simulink model "largeWaterPumpingNetwork"  (R2023b)
settings: Solver=VariableStepAuto  StartTime=0.0  StopTime=200  MaxStep=1  RelTol=1e-5  AbsTol=1e-5  EnableMultiTasking=on
InitFcn:
  | load("largescale_sample.mat")
undefined symbols (not defined in the file or in its folder): input_parameters
libraries: fl_lib x243, nesl_utility x162, SimscapeFluids_lib x129, sdl_lib x40
(part 2 of 12)

== system largeWaterPumpingNetwork/Subsystem 3 ==
  Bus Creator : BusCreator  Inputs=4
  Line 11 : Subsystem  mask{source_pressure=input_parameters.source_pressure_11, pump_speed=input_parameters.pump_speed_11, pipe1_length=input_parameters.pipe1_length_11, pipe2_length=input_parameters.pipe2_length_11, pipe2_ele=input_parameters.pipe2_ele_11}
      mask prompts: source_pressure "Source Pressure (atm)"; pump_speed "Pump Speed (rpm)"; pipe1_length "Pipe #1 Length (m)"; pipe2_length "Pipe #2 Length (m)"; pipe2_ele "PIpe #3 Elevation Gain (m)"
      settings: PortSchema="{\"entries\":[{\"content\":{\"sides\":[{\"content\":{},\"type\":\"ConnectorPlacement.EquallySpacedRectSide\",\"uuid\":\"b3564357-8f52-4949-91c1-42582344ea16\"},{\"content\":{\"connectorIds\":[\"RConn1\"],\"side\":\"RIGHT\"},\"type\":\"ConnectorPlacement.EquallySpacedRectSide\",\"uuid\":\"3df6ff4b-c089-47d9-9218-1d5835660c11\"},{\"content\":{\"connectorIds\":[\"Out1\"],\"side\":\"TOP\"},\"type\":\"ConnectorPlacement.EquallySpacedRectSide\",\"uuid\":\"76d061bd-6b93-4208-81e2-7b97871dfce4\"}]},\"type\":\"ConnectorPlacement.EquallySpacedConnector\",\"uuid\":\"90c8a33d-31fc-4de8-aabb-a154bae7a0ca\"}],\"packageUris\":[\"http://schema.mathworks.com/mf0/Connector/R2020b\"],\"version\":\"1.0\"}"
  Line 12 : Subsystem  mask{source_pressure=input_parameters.source_pressure_12, pump_speed=input_parameters.pump_speed_12, pipe1_length=input_parameters.pipe1_length_12, pipe2_length=input_parameters.pipe2_length_12, pipe2_ele=input_parameters.pipe2_ele_12}
      mask prompts: source_pressure "Source Pressure (atm)"; pump_speed "Pump Speed (rpm)"; pipe1_length "Pipe #1 Length (m)"; pipe2_length "Pipe #2 Length (m)"; pipe2_ele "PIpe #3 Elevation Gain (m)"
      settings: PortSchema="{\"entries\":[{\"content\":{\"sides\":[{\"content\":{},\"type\":\"ConnectorPlacement.EquallySpacedRectSide\",\"uuid\":\"b3564357-8f52-4949-91c1-42582344ea16\"},{\"content\":{\"connectorIds\":[\"RConn1\"],\"side\":\"RIGHT\"},\"type\":\"ConnectorPlacement.EquallySpacedRectSide\",\"uuid\":\"3df6ff4b-c089-47d9-9218-1d5835660c11\"},{\"content\":{\"connectorIds\":[\"Out1\"],\"side\":\"TOP\"},\"type\":\"ConnectorPlacement.EquallySpacedRectSide\",\"uuid\":\"76d061bd-6b93-4208-81e2-7b97871dfce4\"}]},\"type\":\"ConnectorPlacement.EquallySpacedConnector\",\"uuid\":\"90c8a33d-31fc-4de8-aabb-a154bae7a0ca\"}],\"packageUris\":[\"http://schema.mathworks.com/mf0/Connector/R2020b\"],\"version\":\"1.0\"}"
  Line 13 : Subsystem  mask{source_pressure=input_parameters.source_pressure_13, pump_speed=input_parameters.pump_speed_13, pipe1_length=input_parameters.pipe1_length_13, pipe2_length=input_parameters.pipe2_length_13, pipe2_ele=input_parameters.pipe2_ele_13}
      mask prompts: source_pressure "Source Pressure (atm)"; pump_speed "Pump Speed (rpm)"; pipe1_length "Pipe #1 Length (m)"; pipe2_length "Pipe #2 Length (m)"; pipe2_ele "PIpe #3 Elevation Gain (m)"
      settings: PortSchema="{\"entries\":[{\"content\":{\"sides\":[{\"content\":{},\"type\":\"ConnectorPlacement.EquallySpacedRectSide\",\"uuid\":\"b3564357-8f52-4949-91c1-42582344ea16\"},{\"content\":{\"connectorIds\":[\"RConn1\"],\"side\":\"RIGHT\"},\"type\":\"ConnectorPlacement.EquallySpacedRectSide\",\"uuid\":\"3df6ff4b-c089-47d9-9218-1d5835660c11\"},{\"content\":{\"connectorIds\":[\"Out1\"],\"side\":\"TOP\"},\"type\":\"ConnectorPlacement.EquallySpacedRectSide\",\"uuid\":\"76d061bd-6b93-4208-81e2-7b97871dfce4\"}]},\"type\":\"ConnectorPlacement.EquallySpacedConnector\",\"uuid\":\"90c8a33d-31fc-4de8-aabb-a154bae7a0ca\"}],\"packageUris\":[\"http://schema.mathworks.com/mf0/Connector/R2020b\"],\"version\":\"1.0\"}"
  Line 14 : Subsystem  mask{source_pressure=input_parameters.source_pressure_14, pump_speed=input_parameters.pump_speed_14, pipe1_length=input_parameters.pipe1_length_14, pipe2_length=input_parameters.pipe2_length_14, pipe2_ele=input_parameters.pipe2_ele_14}
      mask prompts: source_pressure "Source Pressure (atm)"; pump_speed "Pump Speed (rpm)"; pipe1_length "Pipe #1 Length (m)"; pipe2_length "Pipe #2 Length (m)"; pipe2_ele "PIpe #3 Elevation Gain (m)"
      settings: PortSchema="{\"entries\":[{\"content\":{\"sides\":[{\"content\":{},\"type\":\"ConnectorPlacement.EquallySpacedRectSide\",\"uuid\":\"b3564357-8f52-4949-91c1-42582344ea16\"},{\"content\":{\"connectorIds\":[\"RConn1\"],\"side\":\"RIGHT\"},\"type\":\"ConnectorPlacement.EquallySpacedRectSide\",\"uuid\":\"3df6ff4b-c089-47d9-9218-1d5835660c11\"},{\"content\":{\"connectorIds\":[\"Out1\"],\"side\":\"TOP\"},\"type\":\"ConnectorPlacement.EquallySpacedRectSide\",\"uuid\":\"76d061bd-6b93-4208-81e2-7b97871dfce4\"}]},\"type\":\"ConnectorPlacement.EquallySpacedConnector\",\"uuid\":\"90c8a33d-31fc-4de8-aabb-a154bae7a0ca\"}],\"packageUris\":[\"http://schema.mathworks.com/mf0/Connector/R2020b\"],\"version\":\"1.0\"}"
  Outflow : PMIOPort  Side=Left
  Inflow : PMIOPort  Port=2  Side=Right
  Sensor Signals : Outport
  wires:
  Bus Creator/1 -> Sensor Signals/1  "Sensor Signals"
  [Line11] -> Bus Creator/1  "Line11"
  Line 11/1(Sensor Signals) -> [Line11]
  Line 12/1(Sensor Signals) -> [Line12]
  Line 13/1(Sensor Signals) -> [Line13]
  Line 14/1(Sensor Signals) -> [Line14]
  [Line12] -> Bus Creator/2  "Line12"
  [Line13] -> Bus Creator/3  "Line13"
  [Line14] -> Bus Creator/4  "Line14"
  connections:
  Line 11/RConn1 -- Line 12/RConn1 -- Line 13/RConn1 -- Line 14/RConn1 -- Inflow/RConn1 -- Outflow/RConn1

== system largeWaterPumpingNetwork/Subsystem 4 ==
  Bus Creator : BusCreator  Inputs=5
  Line 15 : Subsystem  mask{source_pressure=input_parameters.source_pressure_15, pump_speed=input_parameters.pump_speed_15, pipe1_length=input_parameters.pipe1_length_15, pipe2_length=input_parameters.pipe2_length_15, pipe2_ele=input_parameters.pipe2_ele_15}
      mask prompts: source_pressure "Source Pressure (atm)"; pump_speed "Pump Speed (rpm)"; pipe1_length "Pipe #1 Length (m)"; pipe2_length "Pipe #2 Length (m)"; pipe2_ele "PIpe #3 Elevation Gain (m)"
      settings: PortSchema="{\"entries\":[{\"content\":{\"sides\":[{\"content\":{},\"type\":\"ConnectorPlacement.EquallySpacedRectSide\",\"uuid\":\"b3564357-8f52-4949-91c1-42582344ea16\"},{\"content\":{\"connectorIds\":[\"RConn1\"],\"side\":\"RIGHT\"},\"type\":\"ConnectorPlacement.EquallySpacedRectSide\",\"uuid\":\"3df6ff4b-c089-47d9-9218-1d5835660c11\"},{\"content\":{\"connectorIds\":[\"Out1\"],\"side\":\"TOP\"},\"type\":\"ConnectorPlacement.EquallySpacedRectSide\",\"uuid\":\"76d061bd-6b93-4208-81e2-7b97871dfce4\"}]},\"type\":\"ConnectorPlacement.EquallySpacedConnector\",\"uuid\":\"90c8a33d-31fc-4de8-aabb-a154bae7a0ca\"}],\"packageUris\":[\"http://schema.mathworks.com/mf0/Connector/R2020b\"],\"version\":\"1.0\"}"
  Line 16 : Subsystem  mask{source_pressure=input_parameters.source_pressure_16, pump_speed=input_parameters.pump_speed_16, pipe1_length=input_parameters.pipe1_length_16, pipe2_length=input_parameters.pipe2_length_16, pipe2_ele=input_parameters.pipe2_ele_16}
      mask prompts: source_pressure "Source Pressure (atm)"; pump_speed "Pump Speed (rpm)"; pipe1_length "Pipe #1 Length (m)"; pipe2_length "Pipe #2 Length (m)"; pipe2_ele "PIpe #3 Elevation Gain (m)"
      settings: PortSchema="{\"entries\":[{\"content\":{\"sides\":[{\"content\":{},\"type\":\"ConnectorPlacement.EquallySpacedRectSide\",\"uuid\":\"b3564357-8f52-4949-91c1-42582344ea16\"},{\"content\":{\"connectorIds\":[\"RConn1\"],\"side\":\"RIGHT\"},\"type\":\"ConnectorPlacement.EquallySpacedRectSide\",\"uuid\":\"3df6ff4b-c089-47d9-9218-1d5835660c11\"},{\"content\":{\"connectorIds\":[\"Out1\"],\"side\":\"TOP\"},\"type\":\"ConnectorPlacement.EquallySpacedRectSide\",\"uuid\":\"76d061bd-6b93-4208-81e2-7b97871dfce4\"}]},\"type\":\"ConnectorPlacement.EquallySpacedConnector\",\"uuid\":\"90c8a33d-31fc-4de8-aabb-a154bae7a0ca\"}],\"packageUris\":[\"http://schema.mathworks.com/mf0/Connector/R2020b\"],\"version\":\"1.0\"}"
  Line 17 : Subsystem  mask{source_pressure=input_parameters.source_pressure_17, pump_speed=input_parameters.pump_speed_17, pipe1_length=input_parameters.pipe1_length_17, pipe2_length=input_parameters.pipe2_length_17, pipe2_ele=input_parameters.pipe2_ele_17}
      mask prompts: source_pressure "Source Pressure (atm)"; pump_speed "Pump Speed (rpm)"; pipe1_length "Pipe #1 Length (m)"; pipe2_length "Pipe #2 Length (m)"; pipe2_ele "PIpe #3 Elevation Gain (m)"
      settings: PortSchema="{\"entries\":[{\"content\":{\"sides\":[{\"content\":{},\"type\":\"ConnectorPlacement.EquallySpacedRectSide\",\"uuid\":\"b3564357-8f52-4949-91c1-42582344ea16\"},{\"content\":{\"connectorIds\":[\"RConn1\"],\"side\":\"RIGHT\"},\"type\":\"ConnectorPlacement.EquallySpacedRectSide\",\"uuid\":\"3df6ff4b-c089-47d9-9218-1d5835660c11\"},{\"content\":{\"connectorIds\":[\"Out1\"],\"side\":\"TOP\"},\"type\":\"ConnectorPlacement.EquallySpacedRectSide\",\"uuid\":\"76d061bd-6b93-4208-81e2-7b97871dfce4\"}]},\"type\":\"ConnectorPlacement.EquallySpacedConnector\",\"uuid\":\"90c8a33d-31fc-4de8-aabb-a154bae7a0ca\"}],\"packageUris\":[\"http://schema.mathworks.com/mf0/Connector/R2020b\"],\"version\":\"1.0\"}"
  Line 18 : Subsystem  mask{source_pressure=input_parameters.source_pressure_18, pump_speed=input_parameters.pump_speed_18, pipe1_length=input_parameters.pipe1_length_18, pipe2_length=input_parameters.pipe2_length_18, pipe2_ele=input_parameters.pipe2_ele_18}
      mask prompts: source_pressure "Source Pressure (atm)"; pump_speed "Pump Speed (rpm)"; pipe1_length "Pipe #1 Length (m)"; pipe2_length "Pipe #2 Length (m)"; pipe2_ele "PIpe #3 Elevation Gain (m)"
      settings: PortSchema="{\"entries\":[{\"content\":{\"sides\":[{\"content\":{},\"type\":\"ConnectorPlacement.EquallySpacedRectSide\",\"uuid\":\"b3564357-8f52-4949-91c1-42582344ea16\"},{\"content\":{\"connectorIds\":[\"RConn1\"],\"side\":\"RIGHT\"},\"type\":\"ConnectorPlacement.EquallySpacedRectSide\",\"uuid\":\"3df6ff4b-c089-47d9-9218-1d5835660c11\"},{\"content\":{\"connectorIds\":[\"Out1\"],\"side\":\"TOP\"},\"type\":\"ConnectorPlacement.EquallySpacedRectSide\",\"uuid\":\"76d061bd-6b93-4208-81e2-7b97871dfce4\"}]},\"type\":\"ConnectorPlacement.EquallySpacedConnector\",\"uuid\":\"90c8a33d-31fc-4de8-aabb-a154bae7a0ca\"}],\"packageUris\":[\"http://schema.mathworks.com/mf0/Connector/R2020b\"],\"version\":\"1.0\"}"
  Line 19 : Subsystem  mask{source_pressure=input_parameters.source_pressure_19, pump_speed=input_parameters.pump_speed_19, pipe1_length=input_parameters.pipe1_length_19, pipe2_length=input_parameters.pipe2_length_19, pipe2_ele=input_parameters.pipe2_ele_19}
      mask prompts: source_pressure "Source Pressure (atm)"; pump_speed "Pump Speed (rpm)"; pipe1_length "Pipe #1 Length (m)"; pipe2_length "Pipe #2 Length (m)"; pipe2_ele "PIpe #3 Elevation Gain (m)"
      settings: PortSchema="{\"entries\":[{\"content\":{\"sides\":[{\"content\":{},\"type\":\"ConnectorPlacement.EquallySpacedRectSide\",\"uuid\":\"b3564357-8f52-4949-91c1-42582344ea16\"},{\"content\":{\"connectorIds\":[\"RConn1\"],\"side\":\"RIGHT\"},\"type\":\"ConnectorPlacement.EquallySpacedRectSide\",\"uuid\":\"3df6ff4b-c089-47d9-9218-1d5835660c11\"},{\"content\":{\"connectorIds\":[\"Out1\"],\"side\":\"TOP\"},\"type\":\"ConnectorPlacement.EquallySpacedRectSide\",\"uuid\":\"76d061bd-6b93-4208-81e2-7b97871dfce4\"}]},\"type\":\"ConnectorPlacement.EquallySpacedConnector\",\"uuid\":\"90c8a33d-31fc-4de8-aabb-a154bae7a0ca\"}],\"packageUris\":[\"http://schema.mathworks.com/mf0/Connector/R2020b\"],\"version\":\"1.0\"}"
  Outflow : PMIOPort  Side=Left
  Inflow : PMIOPort  Port=2  Side=Right
  Sensor Signals : Outport
  wires:
  Bus Creator/1 -> Sensor Signals/1  "Sensor Signals"
  [Line15] -> Bus Creator/1  "Line15"
  Line 15/1(Sensor Signals) -> [Line15]
  Line 16/1(Sensor Signals) -> [Line16]
  Line 17/1(Sensor Signals) -> [Line17]
  Line 18/1(Sensor Signals) -> [Line18]
  [Line16] -> Bus Creator/2  "Line16"
  [Line17] -> Bus Creator/3  "Line17"
  [Line18] -> Bus Creator/4  "Line18"
  Line 19/1(Sensor Signals) -> [Line19]
  [Line19] -> Bus Creator/5  "Line19"
  connections:
  Line 15/RConn1 -- Line 16/RConn1 -- Line 17/RConn1 -- Outflow/RConn1 -- Line 18/RConn1 -- Line 19/RConn1 -- Inflow/RConn1

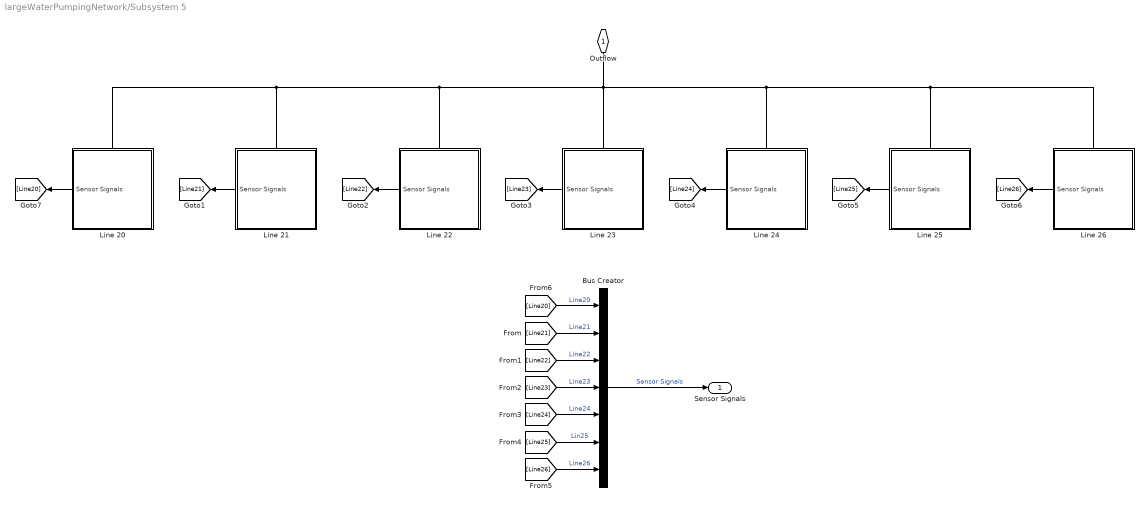
== system largeWaterPumpingNetwork/Subsystem 5 ==
  Bus Creator : BusCreator  Inputs=7
  Line 20 : Subsystem  mask{source_pressure=input_parameters.source_pressure_20, pump_speed=input_parameters.pump_speed_20, pipe1_length=input_parameters.pipe1_length_20, pipe2_length=input_parameters.pipe2_length_20, pipe2_ele=input_parameters.pipe2_ele_20}
      mask prompts: source_pressure "Source Pressure (atm)"; pump_speed "Pump Speed (rpm)"; pipe1_length "Pipe #1 Length (m)"; pipe2_length "Pipe #2 Length (m)"; pipe2_ele "PIpe #3 Elevation Gain (m)"
      settings: PortSchema="{\"entries\":[{\"content\":{\"sides\":[{\"content\":{},\"type\":\"ConnectorPlacement.EquallySpacedRectSide\",\"uuid\":\"b3564357-8f52-4949-91c1-42582344ea16\"},{\"content\":{\"connectorIds\":[\"RConn1\"],\"side\":\"RIGHT\"},\"type\":\"ConnectorPlacement.EquallySpacedRectSide\",\"uuid\":\"3df6ff4b-c089-47d9-9218-1d5835660c11\"},{\"content\":{\"connectorIds\":[\"Out1\"],\"side\":\"TOP\"},\"type\":\"ConnectorPlacement.EquallySpacedRectSide\",\"uuid\":\"76d061bd-6b93-4208-81e2-7b97871dfce4\"}]},\"type\":\"ConnectorPlacement.EquallySpacedConnector\",\"uuid\":\"90c8a33d-31fc-4de8-aabb-a154bae7a0ca\"}],\"packageUris\":[\"http://schema.mathworks.com/mf0/Connector/R2020b\"],\"version\":\"1.0\"}"
  Line 21 : Subsystem  mask{source_pressure=input_parameters.source_pressure_21, pump_speed=input_parameters.pump_speed_21, pipe1_length=input_parameters.pipe1_length_21, pipe2_length=input_parameters.pipe2_length_21, pipe2_ele=input_parameters.pipe2_ele_21}
      mask prompts: source_pressure "Source Pressure (atm)"; pump_speed "Pump Speed (rpm)"; pipe1_length "Pipe #1 Length (m)"; pipe2_length "Pipe #2 Length (m)"; pipe2_ele "PIpe #3 Elevation Gain (m)"
      settings: PortSchema="{\"entries\":[{\"content\":{\"sides\":[{\"content\":{},\"type\":\"ConnectorPlacement.EquallySpacedRectSide\",\"uuid\":\"b3564357-8f52-4949-91c1-42582344ea16\"},{\"content\":{\"connectorIds\":[\"RConn1\"],\"side\":\"RIGHT\"},\"type\":\"ConnectorPlacement.EquallySpacedRectSide\",\"uuid\":\"3df6ff4b-c089-47d9-9218-1d5835660c11\"},{\"content\":{\"connectorIds\":[\"Out1\"],\"side\":\"TOP\"},\"type\":\"ConnectorPlacement.EquallySpacedRectSide\",\"uuid\":\"76d061bd-6b93-4208-81e2-7b97871dfce4\"}]},\"type\":\"ConnectorPlacement.EquallySpacedConnector\",\"uuid\":\"90c8a33d-31fc-4de8-aabb-a154bae7a0ca\"}],\"packageUris\":[\"http://schema.mathworks.com/mf0/Connector/R2020b\"],\"version\":\"1.0\"}"
  Line 22 : Subsystem  mask{source_pressure=input_parameters.source_pressure_22, pump_speed=input_parameters.pump_speed_22, pipe1_length=input_parameters.pipe1_length_22, pipe2_length=input_parameters.pipe2_length_22, pipe2_ele=input_parameters.pipe2_ele_22}
      mask prompts: source_pressure "Source Pressure (atm)"; pump_speed "Pump Speed (rpm)"; pipe1_length "Pipe #1 Length (m)"; pipe2_length "Pipe #2 Length (m)"; pipe2_ele "PIpe #3 Elevation Gain (m)"
      settings: PortSchema="{\"entries\":[{\"content\":{\"sides\":[{\"content\":{},\"type\":\"ConnectorPlacement.EquallySpacedRectSide\",\"uuid\":\"b3564357-8f52-4949-91c1-42582344ea16\"},{\"content\":{\"connectorIds\":[\"RConn1\"],\"side\":\"RIGHT\"},\"type\":\"ConnectorPlacement.EquallySpacedRectSide\",\"uuid\":\"3df6ff4b-c089-47d9-9218-1d5835660c11\"},{\"content\":{\"connectorIds\":[\"Out1\"],\"side\":\"TOP\"},\"type\":\"ConnectorPlacement.EquallySpacedRectSide\",\"uuid\":\"76d061bd-6b93-4208-81e2-7b97871dfce4\"}]},\"type\":\"ConnectorPlacement.EquallySpacedConnector\",\"uuid\":\"90c8a33d-31fc-4de8-aabb-a154bae7a0ca\"}],\"packageUris\":[\"http://schema.mathworks.com/mf0/Connector/R2020b\"],\"version\":\"1.0\"}"
  Line 23 : Subsystem  mask{source_pressure=input_parameters.source_pressure_23, pump_speed=input_parameters.pump_speed_23, pipe1_length=input_parameters.pipe1_length_23, pipe2_length=input_parameters.pipe2_length_23, pipe2_ele=input_parameters.pipe2_ele_23}
      mask prompts: source_pressure "Source Pressure (atm)"; pump_speed "Pump Speed (rpm)"; pipe1_length "Pipe #1 Length (m)"; pipe2_length "Pipe #2 Length (m)"; pipe2_ele "PIpe #3 Elevation Gain (m)"
      settings: PortSchema="{\"entries\":[{\"content\":{\"sides\":[{\"content\":{},\"type\":\"ConnectorPlacement.EquallySpacedRectSide\",\"uuid\":\"b3564357-8f52-4949-91c1-42582344ea16\"},{\"content\":{\"connectorIds\":[\"RConn1\"],\"side\":\"RIGHT\"},\"type\":\"ConnectorPlacement.EquallySpacedRectSide\",\"uuid\":\"3df6ff4b-c089-47d9-9218-1d5835660c11\"},{\"content\":{\"connectorIds\":[\"Out1\"],\"side\":\"TOP\"},\"type\":\"ConnectorPlacement.EquallySpacedRectSide\",\"uuid\":\"76d061bd-6b93-4208-81e2-7b97871dfce4\"}]},\"type\":\"ConnectorPlacement.EquallySpacedConnector\",\"uuid\":\"90c8a33d-31fc-4de8-aabb-a154bae7a0ca\"}],\"packageUris\":[\"http://schema.mathworks.com/mf0/Connector/R2020b\"],\"version\":\"1.0\"}"
  Line 24 : Subsystem  mask{source_pressure=input_parameters.source_pressure_24, pump_speed=input_parameters.pump_speed_24, pipe1_length=input_parameters.pipe1_length_24, pipe2_length=input_parameters.pipe2_length_24, pipe2_ele=input_parameters.pipe2_ele_24}
      mask prompts: source_pressure "Source Pressure (atm)"; pump_speed "Pump Speed (rpm)"; pipe1_length "Pipe #1 Length (m)"; pipe2_length "Pipe #2 Length (m)"; pipe2_ele "PIpe #3 Elevation Gain (m)"
      settings: PortSchema="{\"entries\":[{\"content\":{\"sides\":[{\"content\":{},\"type\":\"ConnectorPlacement.EquallySpacedRectSide\",\"uuid\":\"b3564357-8f52-4949-91c1-42582344ea16\"},{\"content\":{\"connectorIds\":[\"RConn1\"],\"side\":\"RIGHT\"},\"type\":\"ConnectorPlacement.EquallySpacedRectSide\",\"uuid\":\"3df6ff4b-c089-47d9-9218-1d5835660c11\"},{\"content\":{\"connectorIds\":[\"Out1\"],\"side\":\"TOP\"},\"type\":\"ConnectorPlacement.EquallySpacedRectSide\",\"uuid\":\"76d061bd-6b93-4208-81e2-7b97871dfce4\"}]},\"type\":\"ConnectorPlacement.EquallySpacedConnector\",\"uuid\":\"90c8a33d-31fc-4de8-aabb-a154bae7a0ca\"}],\"packageUris\":[\"http://schema.mathworks.com/mf0/Connector/R2020b\"],\"version\":\"1.0\"}"
  Line 25 : Subsystem  mask{source_pressure=input_parameters.source_pressure_25, pump_speed=input_parameters.pump_speed_25, pipe1_length=input_parameters.pipe1_length_25, pipe2_length=input_parameters.pipe2_length_25, pipe2_ele=input_parameters.pipe2_ele_25}
      mask prompts: source_pressure "Source Pressure (atm)"; pump_speed "Pump Speed (rpm)"; pipe1_length "Pipe #1 Length (m)"; pipe2_length "Pipe #2 Length (m)"; pipe2_ele "PIpe #3 Elevation Gain (m)"
      settings: PortSchema="{\"entries\":[{\"content\":{\"sides\":[{\"content\":{},\"type\":\"ConnectorPlacement.EquallySpacedRectSide\",\"uuid\":\"b3564357-8f52-4949-91c1-42582344ea16\"},{\"content\":{\"connectorIds\":[\"RConn1\"],\"side\":\"RIGHT\"},\"type\":\"ConnectorPlacement.EquallySpacedRectSide\",\"uuid\":\"3df6ff4b-c089-47d9-9218-1d5835660c11\"},{\"content\":{\"connectorIds\":[\"Out1\"],\"side\":\"TOP\"},\"type\":\"ConnectorPlacement.EquallySpacedRectSide\",\"uuid\":\"76d061bd-6b93-4208-81e2-7b97871dfce4\"}]},\"type\":\"ConnectorPlacement.EquallySpacedConnector\",\"uuid\":\"90c8a33d-31fc-4de8-aabb-a154bae7a0ca\"}],\"packageUris\":[\"http://schema.mathworks.com/mf0/Connector/R2020b\"],\"version\":\"1.0\"}"
  Line 26 : Subsystem  mask{source_pressure=input_parameters.source_pressure_26, pump_speed=input_parameters.pump_speed_26, pipe1_length=input_parameters.pipe1_length_26, pipe2_length=input_parameters.pipe2_length_26, pipe2_ele=input_parameters.pipe2_ele_26}
      mask prompts: source_pressure "Source Pressure (atm)"; pump_speed "Pump Speed (rpm)"; pipe1_length "Pipe #1 Length (m)"; pipe2_length "Pipe #2 Length (m)"; pipe2_ele "PIpe #3 Elevation Gain (m)"
      settings: PortSchema="{\"entries\":[{\"content\":{\"sides\":[{\"content\":{},\"type\":\"ConnectorPlacement.EquallySpacedRectSide\",\"uuid\":\"b3564357-8f52-4949-91c1-42582344ea16\"},{\"content\":{\"connectorIds\":[\"RConn1\"],\"side\":\"RIGHT\"},\"type\":\"ConnectorPlacement.EquallySpacedRectSide\",\"uuid\":\"3df6ff4b-c089-47d9-9218-1d5835660c11\"},{\"content\":{\"connectorIds\":[\"Out1\"],\"side\":\"TOP\"},\"type\":\"ConnectorPlacement.EquallySpacedRectSide\",\"uuid\":\"76d061bd-6b93-4208-81e2-7b97871dfce4\"}]},\"type\":\"ConnectorPlacement.EquallySpacedConnector\",\"uuid\":\"90c8a33d-31fc-4de8-aabb-a154bae7a0ca\"}],\"packageUris\":[\"http://schema.mathworks.com/mf0/Connector/R2020b\"],\"version\":\"1.0\"}"
  Outflow : PMIOPort  Side=Left
  Sensor Signals : Outport
  wires:
  Bus Creator/1 -> Sensor Signals/1  "Sensor Signals"
  [Line21] -> Bus Creator/2  "Line21"
  Line 21/1(Sensor Signals) -> [Line21]
  Line 22/1(Sensor Signals) -> [Line22]
  Line 23/1(Sensor Signals) -> [Line23]
  Line 24/1(Sensor Signals) -> [Line24]
  [Line22] -> Bus Creator/3  "Line22"
  [Line23] -> Bus Creator/4  "Line23"
  [Line24] -> Bus Creator/5  "Line24"
  Line 25/1(Sensor Signals) -> [Line25]
  Line 26/1(Sensor Signals) -> [Line26]
  [Line25] -> Bus Creator/6  "Lin25"
  [Line26] -> Bus Creator/7  "Line26"
  Line 20/1(Sensor Signals) -> [Line20]
  [Line20] -> Bus Creator/1  "Line20"
  connections:
  Line 20/RConn1 -- Line 21/RConn1 -- Line 22/RConn1 -- Line 23/RConn1 -- Line 24/RConn1 -- Line 25/RConn1 -- Line 26/RConn1 -- Outflow/RConn1

== system largeWaterPumpingNetwork/Subsystem 6 ==
  Bus Creator : BusCreator  Inputs=4
  Line 27 : Subsystem  mask{source_pressure=input_parameters.source_pressure_27, pump_speed=input_parameters.pump_speed_27, pipe1_length=input_parameters.pipe1_length_27, pipe2_length=input_parameters.pipe2_length_27, pipe2_ele=input_parameters.pipe2_ele_27}
      mask prompts: source_pressure "Source Pressure (atm)"; pump_speed "Pump Speed (rpm)"; pipe1_length "Pipe #1 Length (m)"; pipe2_length "Pipe #2 Length (m)"; pipe2_ele "PIpe #3 Elevation Gain (m)"
      settings: PortSchema="{\"entries\":[{\"content\":{\"sides\":[{\"content\":{},\"type\":\"ConnectorPlacement.EquallySpacedRectSide\",\"uuid\":\"b3564357-8f52-4949-91c1-42582344ea16\"},{\"content\":{\"connectorIds\":[\"RConn1\"],\"side\":\"RIGHT\"},\"type\":\"ConnectorPlacement.EquallySpacedRectSide\",\"uuid\":\"3df6ff4b-c089-47d9-9218-1d5835660c11\"},{\"content\":{\"connectorIds\":[\"Out1\"],\"side\":\"TOP\"},\"type\":\"ConnectorPlacement.EquallySpacedRectSide\",\"uuid\":\"76d061bd-6b93-4208-81e2-7b97871dfce4\"}]},\"type\":\"ConnectorPlacement.EquallySpacedConnector\",\"uuid\":\"90c8a33d-31fc-4de8-aabb-a154bae7a0ca\"}],\"packageUris\":[\"http://schema.mathworks.com/mf0/Connector/R2020b\"],\"version\":\"1.0\"}"
  Line 28 : Subsystem  mask{source_pressure=input_parameters.source_pressure_28, pump_speed=input_parameters.pump_speed_28, pipe1_length=input_parameters.pipe1_length_28, pipe2_length=input_parameters.pipe2_length_28, pipe2_ele=input_parameters.pipe2_ele_28}
      mask prompts: source_pressure "Source Pressure (atm)"; pump_speed "Pump Speed (rpm)"; pipe1_length "Pipe #1 Length (m)"; pipe2_length "Pipe #2 Length (m)"; pipe2_ele "PIpe #3 Elevation Gain (m)"
      settings: PortSchema="{\"entries\":[{\"content\":{\"sides\":[{\"content\":{},\"type\":\"ConnectorPlacement.EquallySpacedRectSide\",\"uuid\":\"b3564357-8f52-4949-91c1-42582344ea16\"},{\"content\":{\"connectorIds\":[\"RConn1\"],\"side\":\"RIGHT\"},\"type\":\"ConnectorPlacement.EquallySpacedRectSide\",\"uuid\":\"3df6ff4b-c089-47d9-9218-1d5835660c11\"},{\"content\":{\"connectorIds\":[\"Out1\"],\"side\":\"TOP\"},\"type\":\"ConnectorPlacement.EquallySpacedRectSide\",\"uuid\":\"76d061bd-6b93-4208-81e2-7b97871dfce4\"}]},\"type\":\"ConnectorPlacement.EquallySpacedConnector\",\"uuid\":\"90c8a33d-31fc-4de8-aabb-a154bae7a0ca\"}],\"packageUris\":[\"http://schema.mathworks.com/mf0/Connector/R2020b\"],\"version\":\"1.0\"}"
  Line 29 : Subsystem  mask{source_pressure=input_parameters.source_pressure_29, pump_speed=input_parameters.pump_speed_29, pipe1_length=input_parameters.pipe1_length_29, pipe2_length=input_parameters.pipe2_length_29, pipe2_ele=input_parameters.pipe2_ele_29}
      mask prompts: source_pressure "Source Pressure (atm)"; pump_speed "Pump Speed (rpm)"; pipe1_length "Pipe #1 Length (m)"; pipe2_length "Pipe #2 Length (m)"; pipe2_ele "PIpe #3 Elevation Gain (m)"
      settings: PortSchema="{\"entries\":[{\"content\":{\"sides\":[{\"content\":{},\"type\":\"ConnectorPlacement.EquallySpacedRectSide\",\"uuid\":\"b3564357-8f52-4949-91c1-42582344ea16\"},{\"content\":{\"connectorIds\":[\"RConn1\"],\"side\":\"RIGHT\"},\"type\":\"ConnectorPlacement.EquallySpacedRectSide\",\"uuid\":\"3df6ff4b-c089-47d9-9218-1d5835660c11\"},{\"content\":{\"connectorIds\":[\"Out1\"],\"side\":\"TOP\"},\"type\":\"ConnectorPlacement.EquallySpacedRectSide\",\"uuid\":\"76d061bd-6b93-4208-81e2-7b97871dfce4\"}]},\"type\":\"ConnectorPlacement.EquallySpacedConnector\",\"uuid\":\"90c8a33d-31fc-4de8-aabb-a154bae7a0ca\"}],\"packageUris\":[\"http://schema.mathworks.com/mf0/Connector/R2020b\"],\"version\":\"1.0\"}"
  Line 30 : Subsystem  mask{source_pressure=input_parameters.source_pressure_30, pump_speed=input_parameters.pump_speed_30, pipe1_length=input_parameters.pipe1_length_30, pipe2_length=input_parameters.pipe2_length_30, pipe2_ele=input_parameters.pipe2_ele_30}
      mask prompts: source_pressure "Source Pressure (atm)"; pump_speed "Pump Speed (rpm)"; pipe1_length "Pipe #1 Length (m)"; pipe2_length "Pipe #2 Length (m)"; pipe2_ele "PIpe #3 Elevation Gain (m)"
      settings: PortSchema="{\"entries\":[{\"content\":{\"sides\":[{\"content\":{},\"type\":\"ConnectorPlacement.EquallySpacedRectSide\",\"uuid\":\"b3564357-8f52-4949-91c1-42582344ea16\"},{\"content\":{\"connectorIds\":[\"RConn1\"],\"side\":\"RIGHT\"},\"type\":\"ConnectorPlacement.EquallySpacedRectSide\",\"uuid\":\"3df6ff4b-c089-47d9-9218-1d5835660c11\"},{\"content\":{\"connectorIds\":[\"Out1\"],\"side\":\"TOP\"},\"type\":\"ConnectorPlacement.EquallySpacedRectSide\",\"uuid\":\"76d061bd-6b93-4208-81e2-7b97871dfce4\"}]},\"type\":\"ConnectorPlacement.EquallySpacedConnector\",\"uuid\":\"90c8a33d-31fc-4de8-aabb-a154bae7a0ca\"}],\"packageUris\":[\"http://schema.mathworks.com/mf0/Connector/R2020b\"],\"version\":\"1.0\"}"
  Outflow : PMIOPort  Side=Left
  Sensor Signals : Outport
  wires:
  Bus Creator/1 -> Sensor Signals/1  "Sensor Signals"
  [Line27] -> Bus Creator/1  "Line27"
  Line 27/1(Sensor Signals) -> [Line27]
  Line 28/1(Sensor Signals) -> [Line28]
  Line 29/1(Sensor Signals) -> [Line29]
  Line 30/1(Sensor Signals) -> [Line30]
  [Line28] -> Bus Creator/2  "Line28"
  [Line29] -> Bus Creator/3  "Line29"
  [Line30] -> Bus Creator/4  "Line30"
  connections:
  Line 27/RConn1 -- Line 28/RConn1 -- Line 29/RConn1 -- Line 30/RConn1 -- Outflow/RConn1

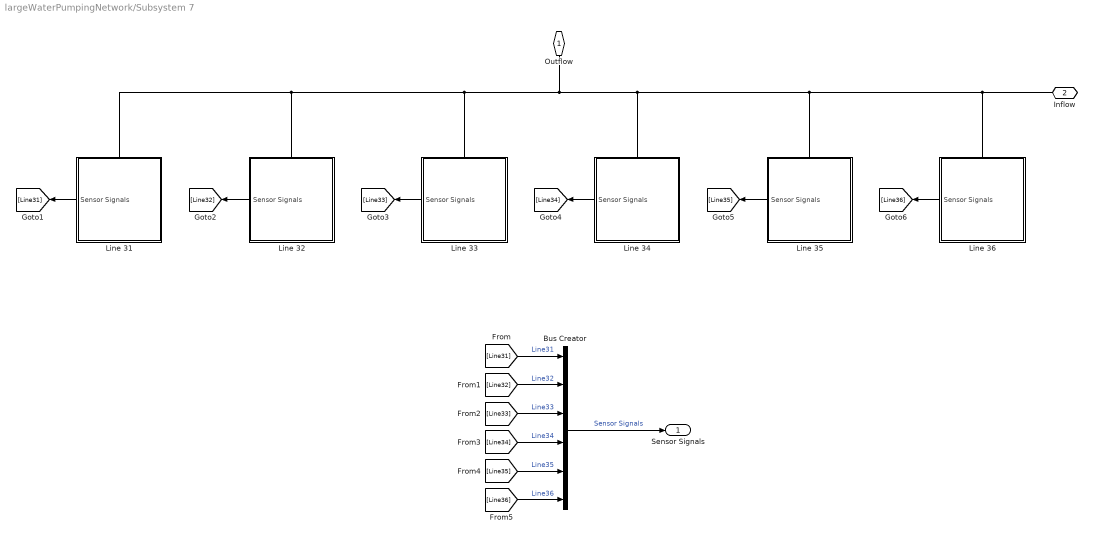
== system largeWaterPumpingNetwork/Subsystem 7 ==
  Bus Creator : BusCreator  Inputs=6
  Line 31 : Subsystem  mask{source_pressure=input_parameters.source_pressure_31, pump_speed=input_parameters.pump_speed_31, pipe1_length=input_parameters.pipe1_length_31, pipe2_length=input_parameters.pipe2_length_31, pipe2_ele=input_parameters.pipe2_ele_31}
      mask prompts: source_pressure "Source Pressure (atm)"; pump_speed "Pump Speed (rpm)"; pipe1_length "Pipe #1 Length (m)"; pipe2_length "Pipe #2 Length (m)"; pipe2_ele "PIpe #3 Elevation Gain (m)"
      settings: PortSchema="{\"entries\":[{\"content\":{\"sides\":[{\"content\":{},\"type\":\"ConnectorPlacement.EquallySpacedRectSide\",\"uuid\":\"b3564357-8f52-4949-91c1-42582344ea16\"},{\"content\":{\"connectorIds\":[\"RConn1\"],\"side\":\"RIGHT\"},\"type\":\"ConnectorPlacement.EquallySpacedRectSide\",\"uuid\":\"3df6ff4b-c089-47d9-9218-1d5835660c11\"},{\"content\":{\"connectorIds\":[\"Out1\"],\"side\":\"TOP\"},\"type\":\"ConnectorPlacement.EquallySpacedRectSide\",\"uuid\":\"76d061bd-6b93-4208-81e2-7b97871dfce4\"}]},\"type\":\"ConnectorPlacement.EquallySpacedConnector\",\"uuid\":\"90c8a33d-31fc-4de8-aabb-a154bae7a0ca\"}],\"packageUris\":[\"http://schema.mathworks.com/mf0/Connector/R2020b\"],\"version\":\"1.0\"}"
  Line 32 : Subsystem  mask{source_pressure=input_parameters.source_pressure_32, pump_speed=input_parameters.pump_speed_32, pipe1_length=input_parameters.pipe1_length_32, pipe2_length=input_parameters.pipe2_length_32, pipe2_ele=input_parameters.pipe2_ele_32}
      mask prompts: source_pressure "Source Pressure (atm)"; pump_speed "Pump Speed (rpm)"; pipe1_length "Pipe #1 Length (m)"; pipe2_length "Pipe #2 Length (m)"; pipe2_ele "PIpe #3 Elevation Gain (m)"
      settings: PortSchema="{\"entries\":[{\"content\":{\"sides\":[{\"content\":{},\"type\":\"ConnectorPlacement.EquallySpacedRectSide\",\"uuid\":\"b3564357-8f52-4949-91c1-42582344ea16\"},{\"content\":{\"connectorIds\":[\"RConn1\"],\"side\":\"RIGHT\"},\"type\":\"ConnectorPlacement.EquallySpacedRectSide\",\"uuid\":\"3df6ff4b-c089-47d9-9218-1d5835660c11\"},{\"content\":{\"connectorIds\":[\"Out1\"],\"side\":\"TOP\"},\"type\":\"ConnectorPlacement.EquallySpacedRectSide\",\"uuid\":\"76d061bd-6b93-4208-81e2-7b97871dfce4\"}]},\"type\":\"ConnectorPlacement.EquallySpacedConnector\",\"uuid\":\"90c8a33d-31fc-4de8-aabb-a154bae7a0ca\"}],\"packageUris\":[\"http://schema.mathworks.com/mf0/Connector/R2020b\"],\"version\":\"1.0\"}"
  Line 33 : Subsystem  mask{source_pressure=input_parameters.source_pressure_33, pump_speed=input_parameters.pump_speed_33, pipe1_length=input_parameters.pipe1_length_33, pipe2_length=input_parameters.pipe2_length_33, pipe2_ele=input_parameters.pipe2_ele_33}
      mask prompts: source_pressure "Source Pressure (atm)"; pump_speed "Pump Speed (rpm)"; pipe1_length "Pipe #1 Length (m)"; pipe2_length "Pipe #2 Length (m)"; pipe2_ele "PIpe #3 Elevation Gain (m)"
      settings: PortSchema="{\"entries\":[{\"content\":{\"sides\":[{\"content\":{},\"type\":\"ConnectorPlacement.EquallySpacedRectSide\",\"uuid\":\"b3564357-8f52-4949-91c1-42582344ea16\"},{\"content\":{\"connectorIds\":[\"RConn1\"],\"side\":\"RIGHT\"},\"type\":\"ConnectorPlacement.EquallySpacedRectSide\",\"uuid\":\"3df6ff4b-c089-47d9-9218-1d5835660c11\"},{\"content\":{\"connectorIds\":[\"Out1\"],\"side\":\"TOP\"},\"type\":\"ConnectorPlacement.EquallySpacedRectSide\",\"uuid\":\"76d061bd-6b93-4208-81e2-7b97871dfce4\"}]},\"type\":\"ConnectorPlacement.EquallySpacedConnector\",\"uuid\":\"90c8a33d-31fc-4de8-aabb-a154bae7a0ca\"}],\"packageUris\":[\"http://schema.mathworks.com/mf0/Connector/R2020b\"],\"version\":\"1.0\"}"
  Line 34 : Subsystem  mask{source_pressure=input_parameters.source_pressure_34, pump_speed=input_parameters.pump_speed_34, pipe1_length=input_parameters.pipe1_length_34, pipe2_length=input_parameters.pipe2_length_34, pipe2_ele=input_parameters.pipe2_ele_34}
      mask prompts: source_pressure "Source Pressure (atm)"; pump_speed "Pump Speed (rpm)"; pipe1_length "Pipe #1 Length (m)"; pipe2_length "Pipe #2 Length (m)"; pipe2_ele "PIpe #3 Elevation Gain (m)"
      settings: PortSchema="{\"entries\":[{\"content\":{\"sides\":[{\"content\":{},\"type\":\"ConnectorPlacement.EquallySpacedRectSide\",\"uuid\":\"b3564357-8f52-4949-91c1-42582344ea16\"},{\"content\":{\"connectorIds\":[\"RConn1\"],\"side\":\"RIGHT\"},\"type\":\"ConnectorPlacement.EquallySpacedRectSide\",\"uuid\":\"3df6ff4b-c089-47d9-9218-1d5835660c11\"},{\"content\":{\"connectorIds\":[\"Out1\"],\"side\":\"TOP\"},\"type\":\"ConnectorPlacement.EquallySpacedRectSide\",\"uuid\":\"76d061bd-6b93-4208-81e2-7b97871dfce4\"}]},\"type\":\"ConnectorPlacement.EquallySpacedConnector\",\"uuid\":\"90c8a33d-31fc-4de8-aabb-a154bae7a0ca\"}],\"packageUris\":[\"http://schema.mathworks.com/mf0/Connector/R2020b\"],\"version\":\"1.0\"}"
  Line 35 : Subsystem  mask{source_pressure=input_parameters.source_pressure_35, pump_speed=input_parameters.pump_speed_35, pipe1_length=input_parameters.pipe1_length_35, pipe2_length=input_parameters.pipe2_length_35, pipe2_ele=input_parameters.pipe2_ele_35}
      mask prompts: source_pressure "Source Pressure (atm)"; pump_speed "Pump Speed (rpm)"; pipe1_length "Pipe #1 Length (m)"; pipe2_length "Pipe #2 Length (m)"; pipe2_ele "PIpe #3 Elevation Gain (m)"
      settings: PortSchema="{\"entries\":[{\"content\":{\"sides\":[{\"content\":{},\"type\":\"ConnectorPlacement.EquallySpacedRectSide\",\"uuid\":\"b3564357-8f52-4949-91c1-42582344ea16\"},{\"content\":{\"connectorIds\":[\"RConn1\"],\"side\":\"RIGHT\"},\"type\":\"ConnectorPlacement.EquallySpacedRectSide\",\"uuid\":\"3df6ff4b-c089-47d9-9218-1d5835660c11\"},{\"content\":{\"connectorIds\":[\"Out1\"],\"side\":\"TOP\"},\"type\":\"ConnectorPlacement.EquallySpacedRectSide\",\"uuid\":\"76d061bd-6b93-4208-81e2-7b97871dfce4\"}]},\"type\":\"ConnectorPlacement.EquallySpacedConnector\",\"uuid\":\"90c8a33d-31fc-4de8-aabb-a154bae7a0ca\"}],\"packageUris\":[\"http://schema.mathworks.com/mf0/Connector/R2020b\"],\"version\":\"1.0\"}"
  Line 36 : Subsystem  mask{source_pressure=input_parameters.source_pressure_36, pump_speed=input_parameters.pump_speed_36, pipe1_length=input_parameters.pipe1_length_36, pipe2_length=input_parameters.pipe2_length_36, pipe2_ele=input_parameters.pipe2_ele_36}
      mask prompts: source_pressure "Source Pressure (atm)"; pump_speed "Pump Speed (rpm)"; pipe1_length "Pipe #1 Length (m)"; pipe2_length "Pipe #2 Length (m)"; pipe2_ele "PIpe #3 Elevation Gain (m)"
      settings: PortSchema="{\"entries\":[{\"content\":{\"sides\":[{\"content\":{},\"type\":\"ConnectorPlacement.EquallySpacedRectSide\",\"uuid\":\"b3564357-8f52-4949-91c1-42582344ea16\"},{\"content\":{\"connectorIds\":[\"RConn1\"],\"side\":\"RIGHT\"},\"type\":\"ConnectorPlacement.EquallySpacedRectSide\",\"uuid\":\"3df6ff4b-c089-47d9-9218-1d5835660c11\"},{\"content\":{\"connectorIds\":[\"Out1\"],\"side\":\"TOP\"},\"type\":\"ConnectorPlacement.EquallySpacedRectSide\",\"uuid\":\"76d061bd-6b93-4208-81e2-7b97871dfce4\"}]},\"type\":\"ConnectorPlacement.EquallySpacedConnector\",\"uuid\":\"90c8a33d-31fc-4de8-aabb-a154bae7a0ca\"}],\"packageUris\":[\"http://schema.mathworks.com/mf0/Connector/R2020b\"],\"version\":\"1.0\"}"
  Outflow : PMIOPort  Side=Left
  Inflow : PMIOPort  Port=2  Side=Right
  Sensor Signals : Outport
  wires:
  Bus Creator/1 -> Sensor Signals/1  "Sensor Signals"
  [Line31] -> Bus Creator/1  "Line31"
  Line 31/1(Sensor Signals) -> [Line31]
  Line 32/1(Sensor Signals) -> [Line32]
  Line 33/1(Sensor Signals) -> [Line33]
  Line 34/1(Sensor Signals) -> [Line34]
  [Line32] -> Bus Creator/2  "Line32"
  [Line33] -> Bus Creator/3  "Line33"
  [Line34] -> Bus Creator/4  "Line34"
  Line 35/1(Sensor Signals) -> [Line35]
  Line 36/1(Sensor Signals) -> [Line36]
  [Line35] -> Bus Creator/5  "Line35"
  [Line36] -> Bus Creator/6  "Line36"
  connections:
  Line 31/RConn1 -- Line 32/RConn1 -- Line 33/RConn1 -- Line 34/RConn1 -- Line 35/RConn1 -- Line 36/RConn1 -- Inflow/RConn1 -- Outflow/RConn1

== system largeWaterPumpingNetwork/Subsystem 8 ==
  Bus Creator : BusCreator  Inputs=4
  Line 37 : Subsystem  mask{source_pressure=input_parameters.source_pressure_37, pump_speed=input_parameters.pump_speed_37, pipe1_length=input_parameters.pipe1_length_37, pipe2_length=input_parameters.pipe2_length_37, pipe2_ele=input_parameters.pipe2_ele_37}
      mask prompts: source_pressure "Source Pressure (atm)"; pump_speed "Pump Speed (rpm)"; pipe1_length "Pipe #1 Length (m)"; pipe2_length "Pipe #2 Length (m)"; pipe2_ele "PIpe #3 Elevation Gain (m)"
      settings: PortSchema="{\"entries\":[{\"content\":{\"sides\":[{\"content\":{},\"type\":\"ConnectorPlacement.EquallySpacedRectSide\",\"uuid\":\"b3564357-8f52-4949-91c1-42582344ea16\"},{\"content\":{\"connectorIds\":[\"RConn1\"],\"side\":\"RIGHT\"},\"type\":\"ConnectorPlacement.EquallySpacedRectSide\",\"uuid\":\"3df6ff4b-c089-47d9-9218-1d5835660c11\"},{\"content\":{\"connectorIds\":[\"Out1\"],\"side\":\"TOP\"},\"type\":\"ConnectorPlacement.EquallySpacedRectSide\",\"uuid\":\"76d061bd-6b93-4208-81e2-7b97871dfce4\"}]},\"type\":\"ConnectorPlacement.EquallySpacedConnector\",\"uuid\":\"90c8a33d-31fc-4de8-aabb-a154bae7a0ca\"}],\"packageUris\":[\"http://schema.mathworks.com/mf0/Connector/R2020b\"],\"version\":\"1.0\"}"
  Line 38 : Subsystem  mask{source_pressure=input_parameters.source_pressure_38, pump_speed=input_parameters.pump_speed_38, pipe1_length=input_parameters.pipe1_length_38, pipe2_length=input_parameters.pipe2_length_38, pipe2_ele=input_parameters.pipe2_ele_38}
      mask prompts: source_pressure "Source Pressure (atm)"; pump_speed "Pump Speed (rpm)"; pipe1_length "Pipe #1 Length (m)"; pipe2_length "Pipe #2 Length (m)"; pipe2_ele "PIpe #3 Elevation Gain (m)"
      settings: PortSchema="{\"entries\":[{\"content\":{\"sides\":[{\"content\":{},\"type\":\"ConnectorPlacement.EquallySpacedRectSide\",\"uuid\":\"b3564357-8f52-4949-91c1-42582344ea16\"},{\"content\":{\"connectorIds\":[\"RConn1\"],\"side\":\"RIGHT\"},\"type\":\"ConnectorPlacement.EquallySpacedRectSide\",\"uuid\":\"3df6ff4b-c089-47d9-9218-1d5835660c11\"},{\"content\":{\"connectorIds\":[\"Out1\"],\"side\":\"TOP\"},\"type\":\"ConnectorPlacement.EquallySpacedRectSide\",\"uuid\":\"76d061bd-6b93-4208-81e2-7b97871dfce4\"}]},\"type\":\"ConnectorPlacement.EquallySpacedConnector\",\"uuid\":\"90c8a33d-31fc-4de8-aabb-a154bae7a0ca\"}],\"packageUris\":[\"http://schema.mathworks.com/mf0/Connector/R2020b\"],\"version\":\"1.0\"}"
  Line 39 : Subsystem  mask{source_pressure=input_parameters.source_pressure_39, pump_speed=input_parameters.pump_speed_39, pipe1_length=input_parameters.pipe1_length_39, pipe2_length=input_parameters.pipe2_length_39, pipe2_ele=input_parameters.pipe2_ele_39}
      mask prompts: source_pressure "Source Pressure (atm)"; pump_speed "Pump Speed (rpm)"; pipe1_length "Pipe #1 Length (m)"; pipe2_length "Pipe #2 Length (m)"; pipe2_ele "PIpe #3 Elevation Gain (m)"
      settings: PortSchema="{\"entries\":[{\"content\":{\"sides\":[{\"content\":{},\"type\":\"ConnectorPlacement.EquallySpacedRectSide\",\"uuid\":\"b3564357-8f52-4949-91c1-42582344ea16\"},{\"content\":{\"connectorIds\":[\"RConn1\"],\"side\":\"RIGHT\"},\"type\":\"ConnectorPlacement.EquallySpacedRectSide\",\"uuid\":\"3df6ff4b-c089-47d9-9218-1d5835660c11\"},{\"content\":{\"connectorIds\":[\"Out1\"],\"side\":\"TOP\"},\"type\":\"ConnectorPlacement.EquallySpacedRectSide\",\"uuid\":\"76d061bd-6b93-4208-81e2-7b97871dfce4\"}]},\"type\":\"ConnectorPlacement.EquallySpacedConnector\",\"uuid\":\"90c8a33d-31fc-4de8-aabb-a154bae7a0ca\"}],\"packageUris\":[\"http://schema.mathworks.com/mf0/Connector/R2020b\"],\"version\":\"1.0\"}"
  Line 40 : Subsystem  mask{source_pressure=input_parameters.source_pressure_40, pump_speed=input_parameters.pump_speed_40, pipe1_length=input_parameters.pipe1_length_40, pipe2_length=input_parameters.pipe2_length_40, pipe2_ele=input_parameters.pipe2_ele_40}
      mask prompts: source_pressure "Source Pressure (atm)"; pump_speed "Pump Speed (rpm)"; pipe1_length "Pipe #1 Length (m)"; pipe2_length "Pipe #2 Length (m)"; pipe2_ele "PIpe #3 Elevation Gain (m)"
      settings: PortSchema="{\"entries\":[{\"content\":{\"sides\":[{\"content\":{},\"type\":\"ConnectorPlacement.EquallySpacedRectSide\",\"uuid\":\"b3564357-8f52-4949-91c1-42582344ea16\"},{\"content\":{\"connectorIds\":[\"RConn1\"],\"side\":\"RIGHT\"},\"type\":\"ConnectorPlacement.EquallySpacedRectSide\",\"uuid\":\"3df6ff4b-c089-47d9-9218-1d5835660c11\"},{\"content\":{\"connectorIds\":[\"Out1\"],\"side\":\"TOP\"},\"type\":\"ConnectorPlacement.EquallySpacedRectSide\",\"uuid\":\"76d061bd-6b93-4208-81e2-7b97871dfce4\"}]},\"type\":\"ConnectorPlacement.EquallySpacedConnector\",\"uuid\":\"90c8a33d-31fc-4de8-aabb-a154bae7a0ca\"}],\"packageUris\":[\"http://schema.mathworks.com/mf0/Connector/R2020b\"],\"version\":\"1.0\"}"
  Outflow : PMIOPort  Side=Left
  Sensor Signals : Outport
  wires:
  Bus Creator/1 -> Sensor Signals/1  "Sensor Signals"
  [Line37] -> Bus Creator/1  "Line37"
  Line 37/1(Sensor Signals) -> [Line37]
  Line 38/1(Sensor Signals) -> [Line38]
  Line 39/1(Sensor Signals) -> [Line39]
  Line 40/1(Sensor Signals) -> [Line40]
  [Line38] -> Bus Creator/2  "Line38"
  [Line39] -> Bus Creator/3  "Line39"
  [Line40] -> Bus Creator/4  "Line40"
  connections:
  Line 38/RConn1 -- Line 37/RConn1 -- Line 40/RConn1 -- Line 39/RConn1 -- Outflow/RConn1
